simulink library "INT_ECBtn_VD"  (R2016b)
settings: Solver=VariableStepAuto  StartTime=0.0  StopTime=10.0  RelTol=1e-3
settings Model: Creator=xinchangran  LastModifiedBy=xinchangran

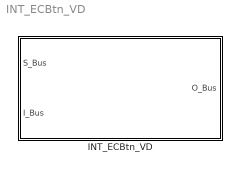
== system INT_ECBtn_VD ==
  INT_ECBtn_VD : Subsystem

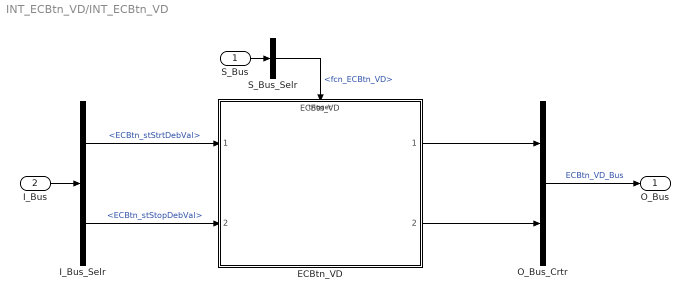
== system INT_ECBtn_VD/INT_ECBtn_VD ==
  S_Bus : Inport
  I_Bus : Inport  Port=2
  ECBtn_VD : ModelReference  ModelNameDialog=ECBtn_VD  SimulationMode=Normal  ModelReferenceVersion=1.11  TriggerPortName=function  TriggerPortTriggerType=function-call  TriggerPortStatesWhenEnabling=held
  I_Bus_Selr : BusSelector  OutputSignals=ECBtn_stStrtDebVal,ECBtn_stStopDebVal
  O_Bus_Crtr : BusCreator  Inputs=2
  S_Bus_Selr : BusSelector  OutputSignals=fcn_ECBtn_VD
  O_Bus : Outport
  wires:
  S_Bus_Selr/1 -> ECBtn_VD/Trigger  "<fcn_ECBtn_VD>"
  S_Bus/1 -> S_Bus_Selr/1
  I_Bus/1 -> I_Bus_Selr/1
  I_Bus_Selr/1 -> ECBtn_VD/1  "<ECBtn_stStrtDebVal>"
  I_Bus_Selr/2 -> ECBtn_VD/2  "<ECBtn_stStopDebVal>"
  O_Bus_Crtr/1 -> O_Bus/1  "ECBtn_VD_Bus"
  ECBtn_VD/1 -> O_Bus_Crtr/1
  ECBtn_VD/2 -> O_Bus_Crtr/2
